simulink model "Ex_2_2"  (R2016b)
settings: Solver=VariableStepAuto  StartTime=0.0  StopTime=10.0  RelTol=1e-3
libraries: Rayannik x3
settings Model: Creator=Alireza7  LastModifiedBy=Alireza7

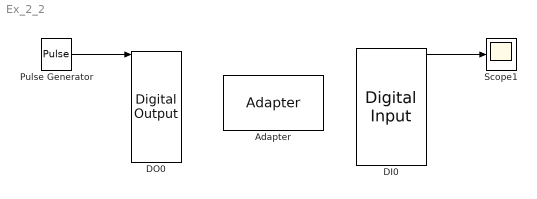
== system Ex_2_2 ==
  Adapter : Rayannik/Adapter  SystemSampleTime=-1
      link override Packet Input1: SampleTime=Ts  MaxMissedTicks=1000000  ShowMissedTicks=off  YieldWhenWaiting=off  DrvName=Standard_Devices/Serial_Port  DrvAddress=3  DrvOptions=[9600 8 0 0 0 0 0 0]  PacketSize=33  DataTypes='33*uint8'  ShowReady=off  ShowError=off  PacketID=1  ByteOrder=1  ShowTimestamp=off
      link override Packet Output1: SampleTime=Ts  MaxMissedTicks=10000000  ShowMissedTicks=off  YieldWhenWaiting=off  DrvName=Standard_Devices/Serial_Port  DrvAddress=3  DrvOptions=[9600 8 0 0 0 0 0 0]  PacketSize=31  DataTypes='31*uint8'  ShowReady=off  ShowError=off  PacketID=1  ByteOrder=1  InitialValue=[]  FinalValue=[]
  DI0 : Rayannik/Digital Input  Priority=2
  DO0 : Rayannik/Digital Output  Priority=2
  Pulse Generator : DiscretePulseGenerator  PulseType=Time based  Amplitude=5  PulseWidth=50
  Scope1 : Scope
  wires:
  DI0/1 -> Scope1/1
  Pulse Generator/1 -> DO0/1
